simulink library "xrbsComm_r3"  (Simulink 5.1)
libraries: xbsIndex_r3 x775, xrbsComm_r3 x1
(part 2 of 6)

== system xrbsComm_r3/White Gaussian  Noise Generator/Box-Muller1/f/lfsr_41_2 ==
  note: 4-Bit Leap-Forward LFSR G(X) = X^41 + X^3 + 1
  reset : Inport
  Concat : xbsIndex_r3/Concat  explicit_period=off  period=1  dbl_ovrd=off
  Concat1 : xbsIndex_r3/Concat  explicit_period=off  period=1  dbl_ovrd=off
  Concat2 : xbsIndex_r3/Concat  explicit_period=off  period=1  dbl_ovrd=off
  Logical{,1..3} (4 alike) : xbsIndex_r3/Logical  logical_function=XOR  inputs=2  precision=User Defined  arith_type=Unsigned  n_bits=1  bin_pt=0  align_bp=on  latency=0  explicit_period=on  period=-1  en=off  dbl_ovrd=off
      settings: xl_area=[0, 0, 0, 0, 0, 0, 0]
  x : xbsIndex_r3/Register  init=init(1)  reg_only_valid=off  explicit_period=off  period=1  rst=on  en=off  out_en=off  dbl_ovrd=off
      settings: xl_area=[0, 0, 0, 0, 0, 0, 0]
  x1 : Subsystem  mask{init=init(6:4:38)}
  x2 : xbsIndex_r3/Register  init=init(2)  reg_only_valid=off  explicit_period=off  period=1  rst=on  en=off  out_en=off  dbl_ovrd=off
      settings: xl_area=[0, 0, 0, 0, 0, 0, 0]
  x3 : xbsIndex_r3/Register  init=init(3)  reg_only_valid=off  explicit_period=off  period=1  rst=on  en=off  out_en=off  dbl_ovrd=off
      settings: xl_area=[0, 0, 0, 0, 0, 0, 0]
  x4 : xbsIndex_r3/Register  init=init(4)  reg_only_valid=off  explicit_period=off  period=1  rst=on  en=off  out_en=off  dbl_ovrd=off
      settings: xl_area=[0, 0, 0, 0, 0, 0, 0]
  x5 : Subsystem  mask{init=init(5:4:41)}
  x6 : Subsystem  mask{init=init(7:4:39)}
  x7 : Subsystem  mask{init=init(8:4:40)}
  " " : Outport
  wires:
  Logical/1 -> x5/1(" ")
  Logical1/1 -> x1/1(" ")
  Logical2/1 -> x6/1(" ")
  Logical3/1 -> x7/1(" ")
  x5/1(z-10) -> x/1, Logical2/2
  x1/1(z-9) -> x2/1, Logical3/2
  x6/1(z-9) -> x3/1, Logical/2
  x7/1(z-9) -> x4/1
  x/1 -> Logical1/1, Concat/1
  x2/1 -> Concat/2, Logical2/1
  Concat/1 -> Concat2/1
  x3/1 -> Concat1/1, Logical3/1
  x4/1 -> Concat1/2, Logical1/2, Logical/1
  Concat1/1 -> Concat2/2
  Concat2/1 -> " "/1
  reset/1 -> x5/2(reset), x1/2(reset), x6/2(reset), x7/2(reset), x/2, x2/2, x3/2, x4/2

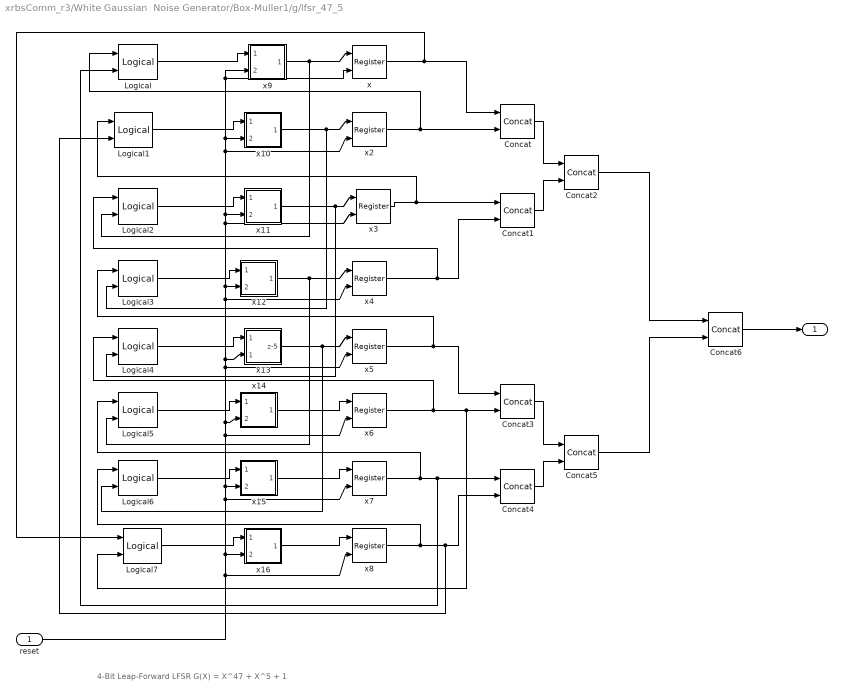
== system xrbsComm_r3/White Gaussian  Noise Generator/Box-Muller1/g/lfsr_47_5 ==
  note: 4-Bit Leap-Forward LFSR G(X) = X^47 + X^5 + 1
  reset : Inport
  Concat{,1..6} (7 alike) : xbsIndex_r3/Concat  explicit_period=off  period=1  dbl_ovrd=off
  Logical{,1..7} (8 alike) : xbsIndex_r3/Logical  logical_function=XOR  inputs=2  precision=User Defined  arith_type=Unsigned  n_bits=1  bin_pt=0  align_bp=on  latency=0  explicit_period=on  period=-1  en=off  dbl_ovrd=off
      settings: xl_area=[0, 0, 0, 0, 0, 0, 0]
  x : xbsIndex_r3/Register  init=init(1)  reg_only_valid=off  explicit_period=off  period=1  rst=on  en=off  out_en=off  dbl_ovrd=off
      settings: xl_area=[0, 0, 0, 0, 0, 0, 0]
  x10 : Subsystem  mask{init=init(10:8:42)}
  x11 : Subsystem  mask{init=init(11:8:43)}
  x12 : Subsystem  mask{init=init(12:8:44)}
  x13 : Subsystem  mask{init=init(13:8:45)}
  x14 : Subsystem  mask{init=init(14:8:46)}
  x15 : Subsystem  mask{init=init(15:8:47)}
  x16 : Subsystem  mask{init=init(16:8:40)}
  x2 : xbsIndex_r3/Register  init=init(2)  reg_only_valid=off  explicit_period=off  period=1  rst=on  en=off  out_en=off  dbl_ovrd=off
      settings: xl_area=[0, 0, 0, 0, 0, 0, 0]
  x3 : xbsIndex_r3/Register  init=init(3)  reg_only_valid=off  explicit_period=off  period=1  rst=on  en=off  out_en=off  dbl_ovrd=off
      settings: xl_area=[0, 0, 0, 0, 0, 0, 0]
  x4 : xbsIndex_r3/Register  init=init(4)  reg_only_valid=off  explicit_period=off  period=1  rst=on  en=off  out_en=off  dbl_ovrd=off
      settings: xl_area=[0, 0, 0, 0, 0, 0, 0]
  x5 : xbsIndex_r3/Register  init=init(5)  reg_only_valid=off  explicit_period=off  period=1  rst=on  en=off  out_en=off  dbl_ovrd=off
      settings: xl_area=[0, 0, 0, 0, 0, 0, 0]
  x6 : xbsIndex_r3/Register  init=init(6)  reg_only_valid=off  explicit_period=off  period=1  rst=on  en=off  out_en=off  dbl_ovrd=off
      settings: xl_area=[0, 0, 0, 0, 0, 0, 0]
  x7 : xbsIndex_r3/Register  init=init(7)  reg_only_valid=off  explicit_period=off  period=1  rst=on  en=off  out_en=off  dbl_ovrd=off
      settings: xl_area=[0, 0, 0, 0, 0, 0, 0]
  x8 : xbsIndex_r3/Register  init=init(8)  reg_only_valid=off  explicit_period=off  period=1  rst=on  en=off  out_en=off  dbl_ovrd=off
      settings: xl_area=[0, 0, 0, 0, 0, 0, 0]
  x9 : Subsystem  mask{init=init(9:8:41)}
  " " : Outport
  wires:
  Logical/1 -> x9/1(" ")
  x9/1(z-5) -> x/1, Logical2/2
  x/1 -> Concat/1, Logical7/1
  x2/1 -> Concat/2, Logical/1
  Concat/1 -> Concat2/1
  x3/1 -> Concat1/1, Logical1/1
  x4/1 -> Concat1/2, Logical2/1
  Concat1/1 -> Concat2/2
  Logical1/1 -> x10/1("  ")
  x10/1(z-5) -> x2/1, Logical3/2
  Logical2/1 -> x11/1(" ")
  x11/1(z-5) -> x3/1, Logical4/2
  Logical3/1 -> x12/1(" ")
  x12/1(z-5) -> x4/1, Logical5/2
  Logical4/1 -> x13/1(" ")
  x13/1(z-5) -> x5/1, Logical6/2
  Logical5/1 -> x14/1(" ")
  x14/1(z-5) -> x6/1
  Logical6/1 -> x15/1(" ")
  x15/1(z-5) -> x7/1
  Logical7/1 -> x16/1(" ")
  x16/1(z-4) -> x8/1
  x6/1 -> Logical4/1, Concat3/2, Logical7/2
  Concat3/1 -> Concat5/1
  Concat4/1 -> Concat5/2
  x5/1 -> Concat3/1, Logical3/1
  x7/1 -> Concat4/1, Logical/2, Logical5/1
  x8/1 -> Concat4/2, Logical1/2, Logical6/1
  Concat2/1 -> Concat6/1
  Concat5/1 -> Concat6/2
  Concat6/1 -> " "/1
  reset/1 -> x9/2(reset), x/2, x10/2(reset), x2/2, x11/2(reset), x3/2, x12/2(reset), x4/2, x13/2(" 1"), x5/2, x14/2(reset), x6/2, x15/2(reset), x7/2, x16/2(reset), x8/2

== system xrbsComm_r3/White Gaussian  Noise Generator/Box-Muller2/fr1/iszero ==
  " " : Inport
  "const " : xbsIndex_r3/Constant  const=0  arith_type=Unsigned  n_bits=4  bin_pt=0  explicit_period=off  period=1  dbl_ovrd=off
  sel1 : xbsIndex_r3/Relational  mode=a=b  latency=1  explicit_period=off  period=1  en=off  dbl_ovrd=off
      settings: xl_area=[0, 0, 0, 0, 0, 0, 0]
  eq : Outport
  wires:
  "const "/1 -> sel1/2
  " "/1 -> sel1/1
  sel1/1 -> eq/1

== system xrbsComm_r3/White Gaussian  Noise Generator/Box-Muller2/fr1/iszero1 ==
  " " : Inport
  Constant1 : xbsIndex_r3/Constant  const=0  arith_type=Unsigned  n_bits=4  bin_pt=0  explicit_period=off  period=1  dbl_ovrd=off
  sel2 : xbsIndex_r3/Relational  mode=a=b  latency=1  explicit_period=off  period=1  en=off  dbl_ovrd=off
      settings: xl_area=[0, 0, 0, 0, 0, 0, 0]
  eq : Outport
  wires:
  Constant1/1 -> sel2/2
  " "/1 -> sel2/1
  sel2/1 -> eq/1

== system xrbsComm_r3/White Gaussian  Noise Generator/Box-Muller2/fr1/iszero2 ==
  " " : Inport
  Constant3 : xbsIndex_r3/Constant  const=0  arith_type=Unsigned  n_bits=4  bin_pt=0  explicit_period=off  period=1  dbl_ovrd=off
  sel3 : xbsIndex_r3/Relational  mode=a=b  latency=1  explicit_period=off  period=1  en=off  dbl_ovrd=off
      settings: xl_area=[0, 0, 0, 0, 0, 0, 0]
  eq : Outport
  wires:
  Constant3/1 -> sel3/2
  " "/1 -> sel3/1
  sel3/1 -> eq/1

== system xrbsComm_r3/White Gaussian  Noise Generator/Box-Muller2/fr1/iszero3 ==
  " " : Inport
  Constant : xbsIndex_r3/Constant  const=0  arith_type=Unsigned  n_bits=4  bin_pt=0  explicit_period=off  period=1  dbl_ovrd=off
  sel4 : xbsIndex_r3/Relational  mode=a=b  latency=1  explicit_period=off  period=1  en=off  dbl_ovrd=off
      settings: xl_area=[0, 0, 0, 0, 0, 0, 0]
  eq : Outport
  wires:
  Constant/1 -> sel4/2
  " "/1 -> sel4/1
  sel4/1 -> eq/1

== system xrbsComm_r3/White Gaussian  Noise Generator/Box-Muller2/fr1/lfsr_17_2 ==
  note: 4-Bit Leap-Forward LFSR G(X) = X^17 + X^3 + 1
  reset : Inport
  Concat : xbsIndex_r3/Concat  explicit_period=off  period=1  dbl_ovrd=off
  Concat1 : xbsIndex_r3/Concat  explicit_period=off  period=1  dbl_ovrd=off
  Concat2 : xbsIndex_r3/Concat  explicit_period=off  period=1  dbl_ovrd=off
  Logical{,1..3} (4 alike) : xbsIndex_r3/Logical  logical_function=XOR  inputs=2  precision=User Defined  arith_type=Unsigned  n_bits=1  bin_pt=0  align_bp=on  latency=0  explicit_period=on  period=-1  en=off  dbl_ovrd=off
      settings: xl_area=[0, 0, 0, 0, 0, 0, 0]
  x : xbsIndex_r3/Register  init=init(1)  reg_only_valid=off  explicit_period=off  period=1  rst=on  en=off  out_en=off  dbl_ovrd=off
      settings: xl_area=[0, 0, 0, 0, 0, 0, 0]
  x1 : Subsystem  mask{init=init(7:4:15)}
  x2 : xbsIndex_r3/Register  init=init(2)  reg_only_valid=off  explicit_period=off  period=1  rst=on  en=off  out_en=off  dbl_ovrd=off
      settings: xl_area=[0, 0, 0, 0, 0, 0, 0]
  x3 : xbsIndex_r3/Register  init=init(3)  reg_only_valid=off  explicit_period=off  period=1  rst=on  en=off  out_en=off  dbl_ovrd=off
      settings: xl_area=[0, 0, 0, 0, 0, 0, 0]
  x4 : xbsIndex_r3/Register  init=init(4)  reg_only_valid=off  explicit_period=off  period=1  rst=on  en=off  out_en=off  dbl_ovrd=off
      settings: xl_area=[0, 0, 0, 0, 0, 0, 0]
  x5 : Subsystem  mask{init=init(5:4:17)}
  x6 : Subsystem  mask{init=init(6:4:14)}
  x7 : Subsystem  mask{init=init(8:4:16)}
  " " : Outport
  wires:
  Logical/1 -> x5/1(" ")
  Logical1/1 -> x6/1(" ")
  Logical2/1 -> x1/1(" ")
  Logical3/1 -> x7/1(" ")
  x5/1(z-4) -> x/1, Logical2/2
  x6/1(z-3) -> x2/1, Logical3/2
  x1/1(z-3) -> x3/1, Logical/2
  x7/1(z-3) -> x4/1
  x/1 -> Logical1/1, Concat/1
  x2/1 -> Concat/2, Logical2/1
  Concat/1 -> Concat2/1
  x3/1 -> Concat1/1, Logical3/1
  x4/1 -> Concat1/2, Logical1/2, Logical/1
  Concat1/1 -> Concat2/2
  Concat2/1 -> " "/1
  reset/1 -> x5/2(reset), x6/2(" reset"), x1/2(" reset"), x7/2(reset), x/2, x2/2, x3/2, x4/2

== system xrbsComm_r3/White Gaussian  Noise Generator/Box-Muller2/fr1/lfsr_25_2 ==
  note: 4-Bit Leap-Forward LFSR G(X) = X^25 + X^3 + 1
  " reset" : Inport
  Concat : xbsIndex_r3/Concat  explicit_period=off  period=1  dbl_ovrd=off
  Concat1 : xbsIndex_r3/Concat  explicit_period=off  period=1  dbl_ovrd=off
  Concat2 : xbsIndex_r3/Concat  explicit_period=off  period=1  dbl_ovrd=off
  Logical{,1..3} (4 alike) : xbsIndex_r3/Logical  logical_function=XOR  inputs=2  precision=User Defined  arith_type=Unsigned  n_bits=1  bin_pt=0  align_bp=on  latency=0  explicit_period=on  period=-1  en=off  dbl_ovrd=off
      settings: xl_area=[0, 0, 0, 0, 0, 0, 0]
  x : xbsIndex_r3/Register  init=init(1)  reg_only_valid=off  explicit_period=off  period=1  rst=on  en=off  out_en=off  dbl_ovrd=off
      settings: xl_area=[0, 0, 0, 0, 0, 0, 0]
  x1 : Subsystem  mask{init=init(7:4:23)}
  x2 : xbsIndex_r3/Register  init=init(2)  reg_only_valid=off  explicit_period=off  period=1  rst=on  en=off  out_en=off  dbl_ovrd=off
      settings: xl_area=[0, 0, 0, 0, 0, 0, 0]
  x3 : xbsIndex_r3/Register  init=init(3)  reg_only_valid=off  explicit_period=off  period=1  rst=on  en=off  out_en=off  dbl_ovrd=off
      settings: xl_area=[0, 0, 0, 0, 0, 0, 0]
  x4 : xbsIndex_r3/Register  init=init(4)  reg_only_valid=off  explicit_period=off  period=1  rst=on  en=off  out_en=off  dbl_ovrd=off
      settings: xl_area=[0, 0, 0, 0, 0, 0, 0]
  x5 : Subsystem  mask{init=init(5:4:25)}
  x6 : Subsystem  mask{init=init(6:4:22)}
  x7 : Subsystem  mask{init=init(8:4:24)}
  " " : Outport
  wires:
  Concat2/1 -> " "/1
  Concat1/1 -> Concat2/2
  x4/1 -> Logical/1, Logical1/2, Concat1/2
  x3/1 -> Logical3/1, Concat1/1
  Concat/1 -> Concat2/1
  x/1 -> Concat/1, Logical1/1
  x7/1(z-5) -> x4/1
  x1/1(z-5) -> Logical/2, x3/1
  x6/1(z-5) -> Logical3/2, x2/1
  x5/1(z-6) -> Logical2/2, x/1
  Logical3/1 -> x7/1(" ")
  Logical2/1 -> x1/1(" ")
  Logical1/1 -> x6/1(" ")
  Logical/1 -> x5/1(" ")
  " reset"/1 -> x7/2(reset), x1/2(reset), x6/2(reset), x5/2(reset), x/2, x2/2, x3/2, x4/2
  x2/1 -> Concat/2, Logical2/1

== system xrbsComm_r3/White Gaussian  Noise Generator/Box-Muller2/fr1/lfsr_29_2 ==
  note: 4-Bit Leap-Forward LFSR G(X) = X^29 + X^2 + 1
  reset : Inport
  Concat : xbsIndex_r3/Concat  explicit_period=off  period=1  dbl_ovrd=off
  Concat1 : xbsIndex_r3/Concat  explicit_period=off  period=1  dbl_ovrd=off
  Concat2 : xbsIndex_r3/Concat  explicit_period=off  period=1  dbl_ovrd=off
  Logical{,1..3} (4 alike) : xbsIndex_r3/Logical  logical_function=XOR  inputs=2  precision=User Defined  arith_type=Unsigned  n_bits=1  bin_pt=0  align_bp=on  latency=0  explicit_period=on  period=-1  en=off  dbl_ovrd=off
      settings: xl_area=[0, 0, 0, 0, 0, 0, 0]
  x : xbsIndex_r3/Register  init=init(1)  reg_only_valid=off  explicit_period=off  period=1  rst=on  en=off  out_en=off  dbl_ovrd=off
      settings: xl_area=[0, 0, 0, 0, 0, 0, 0]
  x2 : xbsIndex_r3/Register  init=init(2)  reg_only_valid=off  explicit_period=off  period=1  rst=on  en=off  out_en=off  dbl_ovrd=off
      settings: xl_area=[0, 0, 0, 0, 0, 0, 0]
  x3 : xbsIndex_r3/Register  init=init(3)  reg_only_valid=off  explicit_period=off  period=1  rst=on  en=off  out_en=off  dbl_ovrd=off
      settings: xl_area=[0, 0, 0, 0, 0, 0, 0]
  x4 : xbsIndex_r3/Register  init=init(4)  reg_only_valid=off  explicit_period=off  period=1  rst=on  en=off  out_en=off  dbl_ovrd=off
      settings: xl_area=[0, 0, 0, 0, 0, 0, 0]
  x5 : Subsystem  mask{init=init(5:4:29)}
  x6 : Subsystem  mask{init=init(6:4:26)}
  x7 : Subsystem  mask{init=init(7:4:27)}
  x8 : Subsystem  mask{init=init(8:4:28)}
  " " : Outport
  wires:
  Logical/1 -> x5/1(" ")
  Logical1/1 -> x6/1(" ")
  Logical2/1 -> x7/1(" ")
  Logical3/1 -> x8/1(" ")
  x5/1(z-7) -> x/1, Logical3/2
  x6/1(z-6) -> x2/1, Logical/2
  x7/1(z-6) -> x3/1
  x8/1(z-6) -> x4/1
  x/1 -> Logical1/1, Concat/1
  x2/1 -> Concat/2, Logical2/1
  Concat/1 -> Concat2/1
  x3/1 -> Concat1/1, Logical1/2, Logical3/1
  x4/1 -> Concat1/2, Logical2/2, Logical/1
  Concat1/1 -> Concat2/2
  Concat2/1 -> " "/1
  reset/1 -> x8/2(reset), x7/2(reset), x6/2(reset), x5/2(reset), x/2, x2/2, x3/2, x4/2

== system xrbsComm_r3/White Gaussian  Noise Generator/Box-Muller2/fr1/lfsr_31_2 ==
  note: 4-Bit Leap-Forward LFSR G(X) = X^31 + X^3 + 1
  reset : Inport
  Concat : xbsIndex_r3/Concat  explicit_period=off  period=1  dbl_ovrd=off
  Concat1 : xbsIndex_r3/Concat  explicit_period=off  period=1  dbl_ovrd=off
  Concat2 : xbsIndex_r3/Concat  explicit_period=off  period=1  dbl_ovrd=off
  Logical{,1..3} (4 alike) : xbsIndex_r3/Logical  logical_function=XOR  inputs=2  precision=User Defined  arith_type=Unsigned  n_bits=1  bin_pt=0  align_bp=on  latency=0  explicit_period=on  period=-1  en=off  dbl_ovrd=off
      settings: xl_area=[0, 0, 0, 0, 0, 0, 0]
  x : xbsIndex_r3/Register  init=init(1)  reg_only_valid=off  explicit_period=off  period=1  rst=on  en=off  out_en=off  dbl_ovrd=off
      settings: xl_area=[0, 0, 0, 0, 0, 0, 0]
  x2 : xbsIndex_r3/Register  init=init(2)  reg_only_valid=off  explicit_period=off  period=1  rst=on  en=off  out_en=off  dbl_ovrd=off
      settings: xl_area=[0, 0, 0, 0, 0, 0, 0]
  x3 : xbsIndex_r3/Register  init=init(3)  reg_only_valid=off  explicit_period=off  period=1  rst=on  en=off  out_en=off  dbl_ovrd=off
      settings: xl_area=[0, 0, 0, 0, 0, 0, 0]
  x4 : xbsIndex_r3/Register  init=init(4)  reg_only_valid=off  explicit_period=off  period=1  rst=on  en=off  out_en=off  dbl_ovrd=off
      settings: xl_area=[0, 0, 0, 0, 0, 0, 0]
  x5 : Subsystem  mask{init=init(5:4:29)}
  x6 : Subsystem  mask{init=init(6:4:30)}
  x7 : Subsystem  mask{init=init(7:4:31)}
  x8 : Subsystem  mask{init=init(8:4:28)}
  " " : Outport
  wires:
  Logical/1 -> x5/1(" ")
  Logical1/1 -> x6/1(" ")
  Logical2/1 -> x7/1(" ")
  Logical3/1 -> x8/1(" ")
  x5/1(z-7) -> Logical/1, x/1
  x6/1(z-7) -> Logical1/1, x2/1
  x7/1(z-7) -> x3/1, Logical2/1
  x8/1(z-6) -> x4/1
  x/1 -> Concat/1, Logical3/1
  x2/1 -> Concat/2, Logical/2
  Concat/1 -> Concat2/1
  x3/1 -> Concat1/1, Logical1/2
  x4/1 -> Logical3/2, Concat1/2, Logical2/2
  Concat1/1 -> Concat2/2
  Concat2/1 -> " "/1
  reset/1 -> x7/2(reset), x5/2(reset), x6/2(reset), x8/2(reset), x/2, x2/2, x3/2, x4/2

== system xrbsComm_r3/White Gaussian  Noise Generator/Box-Muller2/fr1/lfsr_41_2 ==
  note: 4-Bit Leap-Forward LFSR G(X) = X^41 + X^3 + 1
  reset : Inport
  Concat : xbsIndex_r3/Concat  explicit_period=off  period=1  dbl_ovrd=off
  Concat1 : xbsIndex_r3/Concat  explicit_period=off  period=1  dbl_ovrd=off
  Concat2 : xbsIndex_r3/Concat  explicit_period=off  period=1  dbl_ovrd=off
  Logical{,1..3} (4 alike) : xbsIndex_r3/Logical  logical_function=XOR  inputs=2  precision=User Defined  arith_type=Unsigned  n_bits=1  bin_pt=0  align_bp=on  latency=0  explicit_period=on  period=-1  en=off  dbl_ovrd=off
      settings: xl_area=[0, 0, 0, 0, 0, 0, 0]
  x : xbsIndex_r3/Register  init=init(1)  reg_only_valid=off  explicit_period=off  period=1  rst=on  en=off  out_en=off  dbl_ovrd=off
      settings: xl_area=[0, 0, 0, 0, 0, 0, 0]
  x1 : Subsystem  mask{init=init(6:4:38)}
  x2 : xbsIndex_r3/Register  init=init(2)  reg_only_valid=off  explicit_period=off  period=1  rst=on  en=off  out_en=off  dbl_ovrd=off
      settings: xl_area=[0, 0, 0, 0, 0, 0, 0]
  x3 : xbsIndex_r3/Register  init=init(3)  reg_only_valid=off  explicit_period=off  period=1  rst=on  en=off  out_en=off  dbl_ovrd=off
      settings: xl_area=[0, 0, 0, 0, 0, 0, 0]
  x4 : xbsIndex_r3/Register  init=init(4)  reg_only_valid=off  explicit_period=off  period=1  rst=on  en=off  out_en=off  dbl_ovrd=off
      settings: xl_area=[0, 0, 0, 0, 0, 0, 0]
  x5 : Subsystem  mask{init=init(5:4:41)}
  x6 : Subsystem  mask{init=init(7:4:39)}
  x7 : Subsystem  mask{init=init(8:4:40)}
  " " : Outport
  wires:
  Logical/1 -> x5/1(" ")
  Logical1/1 -> x1/1(" ")
  Logical2/1 -> x6/1(" ")
  Logical3/1 -> x7/1(" ")
  x5/1(z-10) -> x/1, Logical2/2
  x1/1(z-9) -> x2/1, Logical3/2
  x6/1(z-9) -> x3/1, Logical/2
  x7/1(z-9) -> x4/1
  x/1 -> Logical1/1, Concat/1
  x2/1 -> Concat/2, Logical2/1
  Concat/1 -> Concat2/1
  x3/1 -> Concat1/1, Logical3/1
  x4/1 -> Concat1/2, Logical1/2, Logical/1
  Concat1/1 -> Concat2/2
  Concat2/1 -> " "/1
  reset/1 -> x5/2(reset), x1/2(reset), x6/2(reset), x7/2(reset), x/2, x2/2, x3/2, x4/2

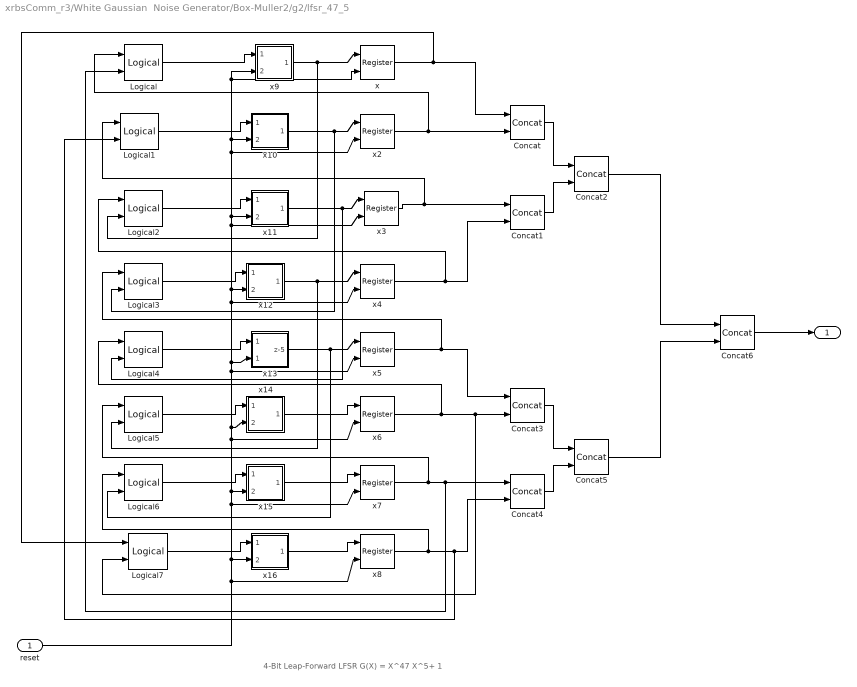
== system xrbsComm_r3/White Gaussian  Noise Generator/Box-Muller2/g2/lfsr_47_5 ==
  note: 4-Bit Leap-Forward LFSR G(X) = X^47 X^5+ 1
  reset : Inport
  Concat{,1..6} (7 alike) : xbsIndex_r3/Concat  explicit_period=off  period=1  dbl_ovrd=off
  Logical{,1..7} (8 alike) : xbsIndex_r3/Logical  logical_function=XOR  inputs=2  precision=User Defined  arith_type=Unsigned  n_bits=1  bin_pt=0  align_bp=on  latency=0  explicit_period=on  period=-1  en=off  dbl_ovrd=off
      settings: xl_area=[0, 0, 0, 0, 0, 0, 0]
  x : xbsIndex_r3/Register  init=init(1)  reg_only_valid=off  explicit_period=off  period=1  rst=on  en=off  out_en=off  dbl_ovrd=off
      settings: xl_area=[0, 0, 0, 0, 0, 0, 0]
  x10 : Subsystem  mask{init=init(10:8:42)}
  x11 : Subsystem  mask{init=init(11:8:43)}
  x12 : Subsystem  mask{init=init(12:8:44)}
  x13 : Subsystem  mask{init=init(13:8:45)}
  x14 : Subsystem  mask{init=init(14:8:46)}
  x15 : Subsystem  mask{init=init(15:8:47)}
  x16 : Subsystem  mask{init=init(16:8:40)}
  x2 : xbsIndex_r3/Register  init=init(2)  reg_only_valid=off  explicit_period=off  period=1  rst=on  en=off  out_en=off  dbl_ovrd=off
      settings: xl_area=[0, 0, 0, 0, 0, 0, 0]
  x3 : xbsIndex_r3/Register  init=init(3)  reg_only_valid=off  explicit_period=off  period=1  rst=on  en=off  out_en=off  dbl_ovrd=off
      settings: xl_area=[0, 0, 0, 0, 0, 0, 0]
  x4 : xbsIndex_r3/Register  init=init(4)  reg_only_valid=off  explicit_period=off  period=1  rst=on  en=off  out_en=off  dbl_ovrd=off
      settings: xl_area=[0, 0, 0, 0, 0, 0, 0]
  x5 : xbsIndex_r3/Register  init=init(5)  reg_only_valid=off  explicit_period=off  period=1  rst=on  en=off  out_en=off  dbl_ovrd=off
      settings: xl_area=[0, 0, 0, 0, 0, 0, 0]
  x6 : xbsIndex_r3/Register  init=init(6)  reg_only_valid=off  explicit_period=off  period=1  rst=on  en=off  out_en=off  dbl_ovrd=off
      settings: xl_area=[0, 0, 0, 0, 0, 0, 0]
  x7 : xbsIndex_r3/Register  init=init(7)  reg_only_valid=off  explicit_period=off  period=1  rst=on  en=off  out_en=off  dbl_ovrd=off
      settings: xl_area=[0, 0, 0, 0, 0, 0, 0]
  x8 : xbsIndex_r3/Register  init=init(8)  reg_only_valid=off  explicit_period=off  period=1  rst=on  en=off  out_en=off  dbl_ovrd=off
      settings: xl_area=[0, 0, 0, 0, 0, 0, 0]
  x9 : Subsystem  mask{init=init(9:8:41)}
  " " : Outport
  wires:
  Logical/1 -> x9/1(" ")
  x9/1(z-5) -> x/1, Logical2/2
  x/1 -> Concat/1, Logical7/1
  x2/1 -> Concat/2, Logical/1
  Concat/1 -> Concat2/1
  x3/1 -> Concat1/1, Logical1/1
  x4/1 -> Concat1/2, Logical2/1
  Concat1/1 -> Concat2/2
  Logical1/1 -> x10/1("  ")
  x10/1(z-5) -> x2/1, Logical3/2
  Logical2/1 -> x11/1(" ")
  x11/1(z-5) -> x3/1, Logical4/2
  Logical3/1 -> x12/1(" ")
  x12/1(z-5) -> x4/1, Logical5/2
  Logical4/1 -> x13/1(" ")
  x13/1(z-5) -> x5/1, Logical6/2
  Logical5/1 -> x14/1(" ")
  x14/1(z-5) -> x6/1
  Logical6/1 -> x15/1(" ")
  x15/1(z-5) -> x7/1
  Logical7/1 -> x16/1(" ")
  x16/1(z-4) -> x8/1
  x6/1 -> Logical4/1, Concat3/2, Logical7/2
  Concat3/1 -> Concat5/1
  Concat4/1 -> Concat5/2
  x5/1 -> Concat3/1, Logical3/1
  x7/1 -> Concat4/1, Logical/2, Logical5/1
  x8/1 -> Concat4/2, Logical1/2, Logical6/1
  Concat2/1 -> Concat6/1
  Concat5/1 -> Concat6/2
  Concat6/1 -> " "/1
  reset/1 -> x9/2(reset), x/2, x10/2(reset), x2/2, x11/2(reset), x3/2, x12/2(reset), x4/2, x13/2(" 1"), x5/2, x14/2(reset), x6/2, x15/2(reset), x7/2, x16/2(reset), x8/2

== system xrbsComm_r3/White Gaussian  Noise Generator/Box-Muller3/fr1/iszero ==
  " " : Inport
  "const " : xbsIndex_r3/Constant  const=0  arith_type=Unsigned  n_bits=4  bin_pt=0  explicit_period=off  period=1  dbl_ovrd=off
  sel1 : xbsIndex_r3/Relational  mode=a=b  latency=1  explicit_period=off  period=1  en=off  dbl_ovrd=off
      settings: xl_area=[0, 0, 0, 0, 0, 0, 0]
  eq : Outport
  wires:
  "const "/1 -> sel1/2
  " "/1 -> sel1/1
  sel1/1 -> eq/1

== system xrbsComm_r3/White Gaussian  Noise Generator/Box-Muller3/fr1/iszero1 ==
  " " : Inport
  Constant1 : xbsIndex_r3/Constant  const=0  arith_type=Unsigned  n_bits=4  bin_pt=0  explicit_period=off  period=1  dbl_ovrd=off
  sel2 : xbsIndex_r3/Relational  mode=a=b  latency=1  explicit_period=off  period=1  en=off  dbl_ovrd=off
      settings: xl_area=[0, 0, 0, 0, 0, 0, 0]
  eq : Outport
  wires:
  Constant1/1 -> sel2/2
  " "/1 -> sel2/1
  sel2/1 -> eq/1

== system xrbsComm_r3/White Gaussian  Noise Generator/Box-Muller3/fr1/iszero2 ==
  " " : Inport
  Constant3 : xbsIndex_r3/Constant  const=0  arith_type=Unsigned  n_bits=4  bin_pt=0  explicit_period=off  period=1  dbl_ovrd=off
  sel3 : xbsIndex_r3/Relational  mode=a=b  latency=1  explicit_period=off  period=1  en=off  dbl_ovrd=off
      settings: xl_area=[0, 0, 0, 0, 0, 0, 0]
  eq : Outport
  wires:
  Constant3/1 -> sel3/2
  " "/1 -> sel3/1
  sel3/1 -> eq/1

== system xrbsComm_r3/White Gaussian  Noise Generator/Box-Muller3/fr1/iszero3 ==
  " " : Inport
  Constant : xbsIndex_r3/Constant  const=0  arith_type=Unsigned  n_bits=4  bin_pt=0  explicit_period=off  period=1  dbl_ovrd=off
  sel4 : xbsIndex_r3/Relational  mode=a=b  latency=1  explicit_period=off  period=1  en=off  dbl_ovrd=off
      settings: xl_area=[0, 0, 0, 0, 0, 0, 0]
  eq : Outport
  wires:
  Constant/1 -> sel4/2
  " "/1 -> sel4/1
  sel4/1 -> eq/1

== system xrbsComm_r3/White Gaussian  Noise Generator/Box-Muller3/fr1/lfsr_17_2 ==
  note: 4-Bit Leap-Forward LFSR G(X) = X^17 + X^3 + 1
  reset : Inport
  Concat : xbsIndex_r3/Concat  explicit_period=off  period=1  dbl_ovrd=off
  Concat1 : xbsIndex_r3/Concat  explicit_period=off  period=1  dbl_ovrd=off
  Concat2 : xbsIndex_r3/Concat  explicit_period=off  period=1  dbl_ovrd=off
  Logical{,1..3} (4 alike) : xbsIndex_r3/Logical  logical_function=XOR  inputs=2  precision=User Defined  arith_type=Unsigned  n_bits=1  bin_pt=0  align_bp=on  latency=0  explicit_period=on  period=-1  en=off  dbl_ovrd=off
      settings: xl_area=[0, 0, 0, 0, 0, 0, 0]
  x : xbsIndex_r3/Register  init=init(1)  reg_only_valid=off  explicit_period=off  period=1  rst=on  en=off  out_en=off  dbl_ovrd=off
      settings: xl_area=[0, 0, 0, 0, 0, 0, 0]
  x1 : Subsystem  mask{init=init(7:4:15)}
  x2 : xbsIndex_r3/Register  init=init(2)  reg_only_valid=off  explicit_period=off  period=1  rst=on  en=off  out_en=off  dbl_ovrd=off
      settings: xl_area=[0, 0, 0, 0, 0, 0, 0]
  x3 : xbsIndex_r3/Register  init=init(3)  reg_only_valid=off  explicit_period=off  period=1  rst=on  en=off  out_en=off  dbl_ovrd=off
      settings: xl_area=[0, 0, 0, 0, 0, 0, 0]
  x4 : xbsIndex_r3/Register  init=init(4)  reg_only_valid=off  explicit_period=off  period=1  rst=on  en=off  out_en=off  dbl_ovrd=off
      settings: xl_area=[0, 0, 0, 0, 0, 0, 0]
  x5 : Subsystem  mask{init=init(5:4:17)}
  x6 : Subsystem  mask{init=init(6:4:14)}
  x7 : Subsystem  mask{init=init(8:4:16)}
  " " : Outport
  wires:
  Logical/1 -> x5/1(" ")
  Logical1/1 -> x6/1(" ")
  Logical2/1 -> x1/1(" ")
  Logical3/1 -> x7/1(" ")
  x5/1(z-4) -> x/1, Logical2/2
  x6/1(z-3) -> x2/1, Logical3/2
  x1/1(z-3) -> x3/1, Logical/2
  x7/1(z-3) -> x4/1
  x/1 -> Logical1/1, Concat/1
  x2/1 -> Concat/2, Logical2/1
  Concat/1 -> Concat2/1
  x3/1 -> Concat1/1, Logical3/1
  x4/1 -> Concat1/2, Logical1/2, Logical/1
  Concat1/1 -> Concat2/2
  Concat2/1 -> " "/1
  reset/1 -> x5/2(reset), x6/2(" reset"), x1/2(" reset"), x7/2(reset), x/2, x2/2, x3/2, x4/2

== system xrbsComm_r3/White Gaussian  Noise Generator/Box-Muller3/fr1/lfsr_25_2 ==
  note: 4-Bit Leap-Forward LFSR G(X) = X^25 + X^3 + 1
  " reset" : Inport
  Concat : xbsIndex_r3/Concat  explicit_period=off  period=1  dbl_ovrd=off
  Concat1 : xbsIndex_r3/Concat  explicit_period=off  period=1  dbl_ovrd=off
  Concat2 : xbsIndex_r3/Concat  explicit_period=off  period=1  dbl_ovrd=off
  Logical{,1..3} (4 alike) : xbsIndex_r3/Logical  logical_function=XOR  inputs=2  precision=User Defined  arith_type=Unsigned  n_bits=1  bin_pt=0  align_bp=on  latency=0  explicit_period=on  period=-1  en=off  dbl_ovrd=off
      settings: xl_area=[0, 0, 0, 0, 0, 0, 0]
  x : xbsIndex_r3/Register  init=init(1)  reg_only_valid=off  explicit_period=off  period=1  rst=on  en=off  out_en=off  dbl_ovrd=off
      settings: xl_area=[0, 0, 0, 0, 0, 0, 0]
  x1 : Subsystem  mask{init=init(7:4:23)}
  x2 : xbsIndex_r3/Register  init=init(2)  reg_only_valid=off  explicit_period=off  period=1  rst=on  en=off  out_en=off  dbl_ovrd=off
      settings: xl_area=[0, 0, 0, 0, 0, 0, 0]
  x3 : xbsIndex_r3/Register  init=init(3)  reg_only_valid=off  explicit_period=off  period=1  rst=on  en=off  out_en=off  dbl_ovrd=off
      settings: xl_area=[0, 0, 0, 0, 0, 0, 0]
  x4 : xbsIndex_r3/Register  init=init(4)  reg_only_valid=off  explicit_period=off  period=1  rst=on  en=off  out_en=off  dbl_ovrd=off
      settings: xl_area=[0, 0, 0, 0, 0, 0, 0]
  x5 : Subsystem  mask{init=init(5:4:25)}
  x6 : Subsystem  mask{init=init(6:4:22)}
  x7 : Subsystem  mask{init=init(8:4:24)}
  " " : Outport
  wires:
  Concat2/1 -> " "/1
  Concat1/1 -> Concat2/2
  x4/1 -> Logical/1, Logical1/2, Concat1/2
  x3/1 -> Logical3/1, Concat1/1
  Concat/1 -> Concat2/1
  x2/1 -> Logical2/1, Concat/2
  x/1 -> Concat/1, Logical1/1
  x7/1(z-5) -> x4/1
  x1/1(z-5) -> Logical/2, x3/1
  x6/1(z-5) -> Logical3/2, x2/1
  x5/1(z-6) -> Logical2/2, x/1
  Logical3/1 -> x7/1(" ")
  Logical2/1 -> x1/1(" ")
  Logical1/1 -> x6/1(" ")
  Logical/1 -> x5/1(" ")
  " reset"/1 -> x7/2(reset), x1/2(reset), x6/2(reset), x5/2(reset), x/2, x2/2, x3/2, x4/2

== system xrbsComm_r3/White Gaussian  Noise Generator/Box-Muller3/fr1/lfsr_29_2 ==
  note: 4-Bit Leap-Forward LFSR G(X) = X^29 + X^2 + 1
  reset : Inport
  Concat : xbsIndex_r3/Concat  explicit_period=off  period=1  dbl_ovrd=off
  Concat1 : xbsIndex_r3/Concat  explicit_period=off  period=1  dbl_ovrd=off
  Concat2 : xbsIndex_r3/Concat  explicit_period=off  period=1  dbl_ovrd=off
  Logical{,1..3} (4 alike) : xbsIndex_r3/Logical  logical_function=XOR  inputs=2  precision=User Defined  arith_type=Unsigned  n_bits=1  bin_pt=0  align_bp=on  latency=0  explicit_period=on  period=-1  en=off  dbl_ovrd=off
      settings: xl_area=[0, 0, 0, 0, 0, 0, 0]
  x : xbsIndex_r3/Register  init=init(1)  reg_only_valid=off  explicit_period=off  period=1  rst=on  en=off  out_en=off  dbl_ovrd=off
      settings: xl_area=[0, 0, 0, 0, 0, 0, 0]
  x2 : xbsIndex_r3/Register  init=init(2)  reg_only_valid=off  explicit_period=off  period=1  rst=on  en=off  out_en=off  dbl_ovrd=off
      settings: xl_area=[0, 0, 0, 0, 0, 0, 0]
  x3 : xbsIndex_r3/Register  init=init(3)  reg_only_valid=off  explicit_period=off  period=1  rst=on  en=off  out_en=off  dbl_ovrd=off
      settings: xl_area=[0, 0, 0, 0, 0, 0, 0]
  x4 : xbsIndex_r3/Register  init=init(4)  reg_only_valid=off  explicit_period=off  period=1  rst=on  en=off  out_en=off  dbl_ovrd=off
      settings: xl_area=[0, 0, 0, 0, 0, 0, 0]
  x5 : Subsystem  mask{init=init(5:4:29)}
  x6 : Subsystem  mask{init=init(6:4:26)}
  x7 : Subsystem  mask{init=init(7:4:27)}
  x8 : Subsystem  mask{init=init(8:4:28)}
  " " : Outport
  wires:
  Logical/1 -> x5/1(" ")
  Logical1/1 -> x6/1(" ")
  Logical2/1 -> x7/1(" ")
  Logical3/1 -> x8/1(" ")
  x5/1(z-7) -> x/1, Logical3/2
  x6/1(z-6) -> x2/1, Logical/2
  x7/1(z-6) -> x3/1
  x8/1(z-6) -> x4/1
  x/1 -> Logical1/1, Concat/1
  x2/1 -> Concat/2, Logical2/1
  Concat/1 -> Concat2/1
  x3/1 -> Concat1/1, Logical1/2, Logical3/1
  x4/1 -> Concat1/2, Logical2/2, Logical/1
  Concat1/1 -> Concat2/2
  Concat2/1 -> " "/1
  reset/1 -> x8/2(reset), x7/2(reset), x6/2(reset), x5/2(reset), x/2, x2/2, x3/2, x4/2

== system xrbsComm_r3/White Gaussian  Noise Generator/Box-Muller3/fr1/lfsr_31_2 ==
  note: 4-Bit Leap-Forward LFSR G(X) = X^31 + X^3 + 1
  reset : Inport
  Concat : xbsIndex_r3/Concat  explicit_period=off  period=1  dbl_ovrd=off
  Concat1 : xbsIndex_r3/Concat  explicit_period=off  period=1  dbl_ovrd=off
  Concat2 : xbsIndex_r3/Concat  explicit_period=off  period=1  dbl_ovrd=off
  Logical{,1..3} (4 alike) : xbsIndex_r3/Logical  logical_function=XOR  inputs=2  precision=User Defined  arith_type=Unsigned  n_bits=1  bin_pt=0  align_bp=on  latency=0  explicit_period=on  period=-1  en=off  dbl_ovrd=off
      settings: xl_area=[0, 0, 0, 0, 0, 0, 0]
  x : xbsIndex_r3/Register  init=init(1)  reg_only_valid=off  explicit_period=off  period=1  rst=on  en=off  out_en=off  dbl_ovrd=off
      settings: xl_area=[0, 0, 0, 0, 0, 0, 0]
  x2 : xbsIndex_r3/Register  init=init(2)  reg_only_valid=off  explicit_period=off  period=1  rst=on  en=off  out_en=off  dbl_ovrd=off
      settings: xl_area=[0, 0, 0, 0, 0, 0, 0]
  x3 : xbsIndex_r3/Register  init=init(3)  reg_only_valid=off  explicit_period=off  period=1  rst=on  en=off  out_en=off  dbl_ovrd=off
      settings: xl_area=[0, 0, 0, 0, 0, 0, 0]
  x4 : xbsIndex_r3/Register  init=init(4)  reg_only_valid=off  explicit_period=off  period=1  rst=on  en=off  out_en=off  dbl_ovrd=off
      settings: xl_area=[0, 0, 0, 0, 0, 0, 0]
  x5 : Subsystem  mask{init=init(5:4:29)}
  x6 : Subsystem  mask{init=init(6:4:30)}
  x7 : Subsystem  mask{init=init(7:4:31)}
  x8 : Subsystem  mask{init=init(8:4:28)}
  " " : Outport
  wires:
  Logical/1 -> x5/1(" ")
  Logical1/1 -> x6/1(" ")
  Logical2/1 -> x7/1(" ")
  Logical3/1 -> x8/1(" ")
  x5/1(z-7) -> Logical/1, x/1
  x6/1(z-7) -> Logical1/1, x2/1
  x7/1(z-7) -> x3/1, Logical2/1
  x8/1(z-6) -> x4/1
  x/1 -> Concat/1, Logical3/1
  x2/1 -> Concat/2, Logical/2
  Concat/1 -> Concat2/1
  x3/1 -> Concat1/1, Logical1/2
  x4/1 -> Logical2/2, Concat1/2, Logical3/2
  Concat1/1 -> Concat2/2
  Concat2/1 -> " "/1
  reset/1 -> x/2, x2/2, x3/2, x4/2, x5/2(reset), x6/2(reset), x7/2(reset), x8/2(reset)

== system xrbsComm_r3/White Gaussian  Noise Generator/Box-Muller3/fr1/lfsr_41_2 ==
  note: 4-Bit Leap-Forward LFSR G(X) = X^41 + X^3 + 1
  reset : Inport
  Concat : xbsIndex_r3/Concat  explicit_period=off  period=1  dbl_ovrd=off
  Concat1 : xbsIndex_r3/Concat  explicit_period=off  period=1  dbl_ovrd=off
  Concat2 : xbsIndex_r3/Concat  explicit_period=off  period=1  dbl_ovrd=off
  Logical{,1..3} (4 alike) : xbsIndex_r3/Logical  logical_function=XOR  inputs=2  precision=User Defined  arith_type=Unsigned  n_bits=1  bin_pt=0  align_bp=on  latency=0  explicit_period=on  period=-1  en=off  dbl_ovrd=off
      settings: xl_area=[0, 0, 0, 0, 0, 0, 0]
  x : xbsIndex_r3/Register  init=init(1)  reg_only_valid=off  explicit_period=off  period=1  rst=on  en=off  out_en=off  dbl_ovrd=off
      settings: xl_area=[0, 0, 0, 0, 0, 0, 0]
  x1 : Subsystem  mask{init=init(6:4:38)}
  x2 : xbsIndex_r3/Register  init=init(2)  reg_only_valid=off  explicit_period=off  period=1  rst=on  en=off  out_en=off  dbl_ovrd=off
      settings: xl_area=[0, 0, 0, 0, 0, 0, 0]
  x3 : xbsIndex_r3/Register  init=init(3)  reg_only_valid=off  explicit_period=off  period=1  rst=on  en=off  out_en=off  dbl_ovrd=off
      settings: xl_area=[0, 0, 0, 0, 0, 0, 0]
  x4 : xbsIndex_r3/Register  init=init(4)  reg_only_valid=off  explicit_period=off  period=1  rst=on  en=off  out_en=off  dbl_ovrd=off
      settings: xl_area=[0, 0, 0, 0, 0, 0, 0]
  x5 : Subsystem  mask{init=init(5:4:41)}
  x6 : Subsystem  mask{init=init(7:4:39)}
  x7 : Subsystem  mask{init=init(8:4:40)}
  " " : Outport
  wires:
  Logical/1 -> x5/1(" ")
  Logical1/1 -> x1/1(" ")
  Logical2/1 -> x6/1(" ")
  Logical3/1 -> x7/1(" ")
  x5/1(z-10) -> x/1, Logical2/2
  x1/1(z-9) -> x2/1, Logical3/2
  x6/1(z-9) -> x3/1, Logical/2
  x7/1(z-9) -> x4/1
  x/1 -> Logical1/1, Concat/1
  x2/1 -> Concat/2, Logical2/1
  Concat/1 -> Concat2/1
  x3/1 -> Concat1/1, Logical3/1
  x4/1 -> Concat1/2, Logical/1, Logical1/2
  Concat1/1 -> Concat2/2
  Concat2/1 -> " "/1
  reset/1 -> x5/2(reset), x1/2(reset), x6/2(reset), x7/2(reset), x/2, x2/2, x3/2, x4/2

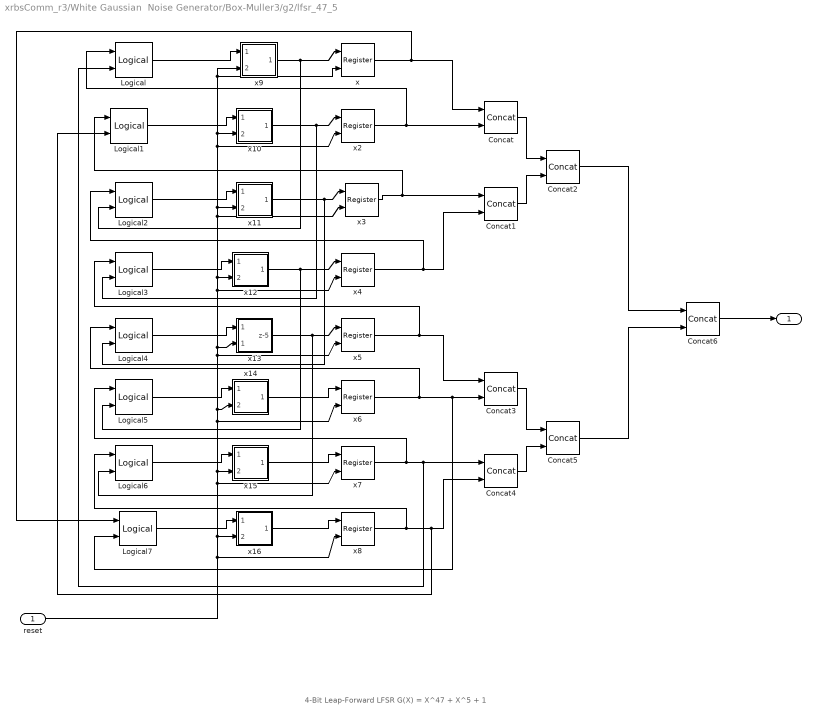
== system xrbsComm_r3/White Gaussian  Noise Generator/Box-Muller3/g2/lfsr_47_5 ==
  note: 4-Bit Leap-Forward LFSR G(X) = X^47 + X^5 + 1
  reset : Inport
  Concat{,1..6} (7 alike) : xbsIndex_r3/Concat  explicit_period=off  period=1  dbl_ovrd=off
  Logical{,1..7} (8 alike) : xbsIndex_r3/Logical  logical_function=XOR  inputs=2  precision=User Defined  arith_type=Unsigned  n_bits=1  bin_pt=0  align_bp=on  latency=0  explicit_period=on  period=-1  en=off  dbl_ovrd=off
      settings: xl_area=[0, 0, 0, 0, 0, 0, 0]
  x : xbsIndex_r3/Register  init=init(1)  reg_only_valid=off  explicit_period=off  period=1  rst=on  en=off  out_en=off  dbl_ovrd=off
      settings: xl_area=[0, 0, 0, 0, 0, 0, 0]
  x10 : Subsystem  mask{init=init(10:8:42)}
  x11 : Subsystem  mask{init=init(11:8:43)}
  x12 : Subsystem  mask{init=init(12:8:44)}
  x13 : Subsystem  mask{init=init(13:8:45)}
  x14 : Subsystem  mask{init=init(14:8:46)}
  x15 : Subsystem  mask{init=init(15:8:47)}
  x16 : Subsystem  mask{init=init(16:8:40)}
  x2 : xbsIndex_r3/Register  init=init(2)  reg_only_valid=off  explicit_period=off  period=1  rst=on  en=off  out_en=off  dbl_ovrd=off
      settings: xl_area=[0, 0, 0, 0, 0, 0, 0]
  x3 : xbsIndex_r3/Register  init=init(3)  reg_only_valid=off  explicit_period=off  period=1  rst=on  en=off  out_en=off  dbl_ovrd=off
      settings: xl_area=[0, 0, 0, 0, 0, 0, 0]
  x4 : xbsIndex_r3/Register  init=init(4)  reg_only_valid=off  explicit_period=off  period=1  rst=on  en=off  out_en=off  dbl_ovrd=off
      settings: xl_area=[0, 0, 0, 0, 0, 0, 0]
  x5 : xbsIndex_r3/Register  init=init(5)  reg_only_valid=off  explicit_period=off  period=1  rst=on  en=off  out_en=off  dbl_ovrd=off
      settings: xl_area=[0, 0, 0, 0, 0, 0, 0]
  x6 : xbsIndex_r3/Register  init=init(6)  reg_only_valid=off  explicit_period=off  period=1  rst=on  en=off  out_en=off  dbl_ovrd=off
      settings: xl_area=[0, 0, 0, 0, 0, 0, 0]
  x7 : xbsIndex_r3/Register  init=init(7)  reg_only_valid=off  explicit_period=off  period=1  rst=on  en=off  out_en=off  dbl_ovrd=off
      settings: xl_area=[0, 0, 0, 0, 0, 0, 0]
  x8 : xbsIndex_r3/Register  init=init(8)  reg_only_valid=off  explicit_period=off  period=1  rst=on  en=off  out_en=off  dbl_ovrd=off
      settings: xl_area=[0, 0, 0, 0, 0, 0, 0]
  x9 : Subsystem  mask{init=init(9:8:41)}
  " " : Outport
  wires:
  Logical/1 -> x9/1(" ")
  x9/1(z-5) -> x/1, Logical2/2
  x/1 -> Concat/1, Logical7/1
  x2/1 -> Concat/2, Logical/1
  Concat/1 -> Concat2/1
  x3/1 -> Concat1/1, Logical1/1
  x4/1 -> Concat1/2, Logical2/1
  Concat1/1 -> Concat2/2
  Logical1/1 -> x10/1("  ")
  x10/1(z-5) -> x2/1, Logical3/2
  Logical2/1 -> x11/1(" ")
  x11/1(z-5) -> x3/1, Logical4/2
  Logical3/1 -> x12/1(" ")
  x12/1(z-5) -> x4/1, Logical5/2
  Logical4/1 -> x13/1(" ")
  x13/1(z-5) -> x5/1, Logical6/2
  Logical5/1 -> x14/1(" ")
  x14/1(z-5) -> x6/1
  Logical6/1 -> x15/1(" ")
  x15/1(z-5) -> x7/1
  Logical7/1 -> x16/1(" ")
  x16/1(z-4) -> x8/1
  x6/1 -> Logical4/1, Concat3/2, Logical7/2
  Concat3/1 -> Concat5/1
  Concat4/1 -> Concat5/2
  x5/1 -> Concat3/1, Logical3/1
  x7/1 -> Concat4/1, Logical/2, Logical5/1
  x8/1 -> Concat4/2, Logical1/2, Logical6/1
  Concat2/1 -> Concat6/1
  Concat5/1 -> Concat6/2
  Concat6/1 -> " "/1
  reset/1 -> x9/2(reset), x/2, x10/2(reset), x2/2, x11/2(reset), x3/2, x12/2(reset), x4/2, x13/2(" 1"), x5/2, x14/2(reset), x6/2, x15/2(reset), x7/2, x16/2(reset), x8/2

== system xrbsComm_r3/White Gaussian  Noise Generator/Box-Muller4/fr1/iszero ==
  " " : Inport
  "const " : xbsIndex_r3/Constant  const=0  arith_type=Unsigned  n_bits=4  bin_pt=0  explicit_period=off  period=1  dbl_ovrd=off
  sel1 : xbsIndex_r3/Relational  mode=a=b  latency=1  explicit_period=off  period=1  en=off  dbl_ovrd=off
      settings: xl_area=[0, 0, 0, 0, 0, 0, 0]
  eq : Outport
  wires:
  "const "/1 -> sel1/2
  " "/1 -> sel1/1
  sel1/1 -> eq/1

== system xrbsComm_r3/White Gaussian  Noise Generator/Box-Muller4/fr1/iszero1 ==
  " " : Inport
  Constant1 : xbsIndex_r3/Constant  const=0  arith_type=Unsigned  n_bits=4  bin_pt=0  explicit_period=off  period=1  dbl_ovrd=off
  sel2 : xbsIndex_r3/Relational  mode=a=b  latency=1  explicit_period=off  period=1  en=off  dbl_ovrd=off
      settings: xl_area=[0, 0, 0, 0, 0, 0, 0]
  eq : Outport
  wires:
  Constant1/1 -> sel2/2
  " "/1 -> sel2/1
  sel2/1 -> eq/1

== system xrbsComm_r3/White Gaussian  Noise Generator/Box-Muller4/fr1/iszero2 ==
  " " : Inport
  Constant3 : xbsIndex_r3/Constant  const=0  arith_type=Unsigned  n_bits=4  bin_pt=0  explicit_period=off  period=1  dbl_ovrd=off
  sel3 : xbsIndex_r3/Relational  mode=a=b  latency=1  explicit_period=off  period=1  en=off  dbl_ovrd=off
      settings: xl_area=[0, 0, 0, 0, 0, 0, 0]
  eq : Outport
  wires:
  Constant3/1 -> sel3/2
  " "/1 -> sel3/1
  sel3/1 -> eq/1

== system xrbsComm_r3/White Gaussian  Noise Generator/Box-Muller4/fr1/iszero3 ==
  " " : Inport
  Constant : xbsIndex_r3/Constant  const=0  arith_type=Unsigned  n_bits=4  bin_pt=0  explicit_period=off  period=1  dbl_ovrd=off
  sel4 : xbsIndex_r3/Relational  mode=a=b  latency=1  explicit_period=off  period=1  en=off  dbl_ovrd=off
      settings: xl_area=[0, 0, 0, 0, 0, 0, 0]
  eq : Outport
  wires:
  Constant/1 -> sel4/2
  " "/1 -> sel4/1
  sel4/1 -> eq/1

== system xrbsComm_r3/White Gaussian  Noise Generator/Box-Muller4/fr1/lfsr_17_2 ==
  note: 4-Bit Leap-Forward LFSR G(X) = X^17 + X^3 + 1
  reset : Inport
  Concat : xbsIndex_r3/Concat  explicit_period=off  period=1  dbl_ovrd=off
  Concat1 : xbsIndex_r3/Concat  explicit_period=off  period=1  dbl_ovrd=off
  Concat2 : xbsIndex_r3/Concat  explicit_period=off  period=1  dbl_ovrd=off
  Logical{,1..3} (4 alike) : xbsIndex_r3/Logical  logical_function=XOR  inputs=2  precision=User Defined  arith_type=Unsigned  n_bits=1  bin_pt=0  align_bp=on  latency=0  explicit_period=on  period=-1  en=off  dbl_ovrd=off
      settings: xl_area=[0, 0, 0, 0, 0, 0, 0]
  x : xbsIndex_r3/Register  init=init(1)  reg_only_valid=off  explicit_period=off  period=1  rst=on  en=off  out_en=off  dbl_ovrd=off
      settings: xl_area=[0, 0, 0, 0, 0, 0, 0]
  x1 : Subsystem  mask{init=init(7:4:15)}
  x2 : xbsIndex_r3/Register  init=init(2)  reg_only_valid=off  explicit_period=off  period=1  rst=on  en=off  out_en=off  dbl_ovrd=off
      settings: xl_area=[0, 0, 0, 0, 0, 0, 0]
  x3 : xbsIndex_r3/Register  init=init(3)  reg_only_valid=off  explicit_period=off  period=1  rst=on  en=off  out_en=off  dbl_ovrd=off
      settings: xl_area=[0, 0, 0, 0, 0, 0, 0]
  x4 : xbsIndex_r3/Register  init=init(4)  reg_only_valid=off  explicit_period=off  period=1  rst=on  en=off  out_en=off  dbl_ovrd=off
      settings: xl_area=[0, 0, 0, 0, 0, 0, 0]
  x5 : Subsystem  mask{init=init(5:4:17)}
  x6 : Subsystem  mask{init=init(6:4:14)}
  x7 : Subsystem  mask{init=init(8:4:16)}
  " " : Outport
  wires:
  Logical/1 -> x5/1(" ")
  Logical1/1 -> x6/1(" ")
  Logical2/1 -> x1/1(" ")
  Logical3/1 -> x7/1(" ")
  x5/1(z-4) -> x/1, Logical2/2
  x6/1(z-3) -> x2/1, Logical3/2
  x1/1(z-3) -> x3/1, Logical/2
  x7/1(z-3) -> x4/1
  x/1 -> Logical1/1, Concat/1
  x2/1 -> Concat/2, Logical2/1
  Concat/1 -> Concat2/1
  x3/1 -> Concat1/1, Logical3/1
  x4/1 -> Concat1/2, Logical1/2, Logical/1
  Concat1/1 -> Concat2/2
  Concat2/1 -> " "/1
  reset/1 -> x5/2(reset), x6/2(" reset"), x1/2(" reset"), x7/2(reset), x/2, x2/2, x3/2, x4/2

== system xrbsComm_r3/White Gaussian  Noise Generator/Box-Muller4/fr1/lfsr_25_2 ==
  note: 4-Bit Leap-Forward LFSR G(X) = X^25 + X^3 + 1
  " reset" : Inport
  Concat : xbsIndex_r3/Concat  explicit_period=off  period=1  dbl_ovrd=off
  Concat1 : xbsIndex_r3/Concat  explicit_period=off  period=1  dbl_ovrd=off
  Concat2 : xbsIndex_r3/Concat  explicit_period=off  period=1  dbl_ovrd=off
  Logical{,1..3} (4 alike) : xbsIndex_r3/Logical  logical_function=XOR  inputs=2  precision=User Defined  arith_type=Unsigned  n_bits=1  bin_pt=0  align_bp=on  latency=0  explicit_period=on  period=-1  en=off  dbl_ovrd=off
      settings: xl_area=[0, 0, 0, 0, 0, 0, 0]
  x : xbsIndex_r3/Register  init=init(1)  reg_only_valid=off  explicit_period=off  period=1  rst=on  en=off  out_en=off  dbl_ovrd=off
      settings: xl_area=[0, 0, 0, 0, 0, 0, 0]
  x1 : Subsystem  mask{init=init(7:4:23)}
  x2 : xbsIndex_r3/Register  init=init(2)  reg_only_valid=off  explicit_period=off  period=1  rst=on  en=off  out_en=off  dbl_ovrd=off
      settings: xl_area=[0, 0, 0, 0, 0, 0, 0]
  x3 : xbsIndex_r3/Register  init=init(3)  reg_only_valid=off  explicit_period=off  period=1  rst=on  en=off  out_en=off  dbl_ovrd=off
      settings: xl_area=[0, 0, 0, 0, 0, 0, 0]
  x4 : xbsIndex_r3/Register  init=init(4)  reg_only_valid=off  explicit_period=off  period=1  rst=on  en=off  out_en=off  dbl_ovrd=off
      settings: xl_area=[0, 0, 0, 0, 0, 0, 0]
  x5 : Subsystem  mask{init=init(5:4:25)}
  x6 : Subsystem  mask{init=init(6:4:22)}
  x7 : Subsystem  mask{init=init(8:4:24)}
  " " : Outport
  wires:
  Concat2/1 -> " "/1
  Concat1/1 -> Concat2/2
  x4/1 -> Logical/1, Logical1/2, Concat1/2
  x3/1 -> Logical3/1, Concat1/1
  Concat/1 -> Concat2/1
  x2/1 -> Logical2/1, Concat/2
  x/1 -> Concat/1, Logical1/1
  x7/1(z-5) -> x4/1
  x1/1(z-5) -> Logical/2, x3/1
  x6/1(z-5) -> Logical3/2, x2/1
  x5/1(z-6) -> Logical2/2, x/1
  Logical3/1 -> x7/1(" ")
  Logical2/1 -> x1/1(" ")
  Logical1/1 -> x6/1(" ")
  Logical/1 -> x5/1(" ")
  " reset"/1 -> x7/2(reset), x1/2(reset), x6/2(reset), x5/2(reset), x/2, x2/2, x3/2, x4/2

== system xrbsComm_r3/White Gaussian  Noise Generator/Box-Muller4/fr1/lfsr_29_2 ==
  note: 4-Bit Leap-Forward LFSR G(X) = X^29 + X^2 + 1
  reset : Inport
  Concat : xbsIndex_r3/Concat  explicit_period=off  period=1  dbl_ovrd=off
  Concat1 : xbsIndex_r3/Concat  explicit_period=off  period=1  dbl_ovrd=off
  Concat2 : xbsIndex_r3/Concat  explicit_period=off  period=1  dbl_ovrd=off
  Logical{,1..3} (4 alike) : xbsIndex_r3/Logical  logical_function=XOR  inputs=2  precision=User Defined  arith_type=Unsigned  n_bits=1  bin_pt=0  align_bp=on  latency=0  explicit_period=on  period=-1  en=off  dbl_ovrd=off
      settings: xl_area=[0, 0, 0, 0, 0, 0, 0]
  x : xbsIndex_r3/Register  init=init(1)  reg_only_valid=off  explicit_period=off  period=1  rst=on  en=off  out_en=off  dbl_ovrd=off
      settings: xl_area=[0, 0, 0, 0, 0, 0, 0]
  x2 : xbsIndex_r3/Register  init=init(2)  reg_only_valid=off  explicit_period=off  period=1  rst=on  en=off  out_en=off  dbl_ovrd=off
      settings: xl_area=[0, 0, 0, 0, 0, 0, 0]
  x3 : xbsIndex_r3/Register  init=init(3)  reg_only_valid=off  explicit_period=off  period=1  rst=on  en=off  out_en=off  dbl_ovrd=off
      settings: xl_area=[0, 0, 0, 0, 0, 0, 0]
  x4 : xbsIndex_r3/Register  init=init(4)  reg_only_valid=off  explicit_period=off  period=1  rst=on  en=off  out_en=off  dbl_ovrd=off
      settings: xl_area=[0, 0, 0, 0, 0, 0, 0]
  x5 : Subsystem  mask{init=init(5:4:29)}
  x6 : Subsystem  mask{init=init(6:4:26)}
  x7 : Subsystem  mask{init=init(7:4:27)}
  x8 : Subsystem  mask{init=init(8:4:28)}
  " " : Outport
  wires:
  Logical/1 -> x5/1(" ")
  Logical1/1 -> x6/1(" ")
  Logical2/1 -> x7/1(" ")
  Logical3/1 -> x8/1(" ")
  x5/1(z-7) -> x/1, Logical3/2
  x6/1(z-6) -> x2/1, Logical/2
  x7/1(z-6) -> x3/1
  x8/1(z-6) -> x4/1
  x/1 -> Logical1/1, Concat/1
  x2/1 -> Concat/2, Logical2/1
  Concat/1 -> Concat2/1
  x3/1 -> Concat1/1, Logical1/2, Logical3/1
  x4/1 -> Concat1/2, Logical2/2, Logical/1
  Concat1/1 -> Concat2/2
  Concat2/1 -> " "/1
  reset/1 -> x8/2(reset), x7/2(reset), x6/2(reset), x5/2(reset), x/2, x2/2, x3/2, x4/2

== system xrbsComm_r3/White Gaussian  Noise Generator/Box-Muller4/fr1/lfsr_31_2 ==
  note: 4-Bit Leap-Forward LFSR G(X) = X^31 + X^3 + 1
  reset : Inport
  Concat : xbsIndex_r3/Concat  explicit_period=off  period=1  dbl_ovrd=off
  Concat1 : xbsIndex_r3/Concat  explicit_period=off  period=1  dbl_ovrd=off
  Concat2 : xbsIndex_r3/Concat  explicit_period=off  period=1  dbl_ovrd=off
  Logical{,1..3} (4 alike) : xbsIndex_r3/Logical  logical_function=XOR  inputs=2  precision=User Defined  arith_type=Unsigned  n_bits=1  bin_pt=0  align_bp=on  latency=0  explicit_period=on  period=-1  en=off  dbl_ovrd=off
      settings: xl_area=[0, 0, 0, 0, 0, 0, 0]
  x : xbsIndex_r3/Register  init=init(1)  reg_only_valid=off  explicit_period=off  period=1  rst=on  en=off  out_en=off  dbl_ovrd=off
      settings: xl_area=[0, 0, 0, 0, 0, 0, 0]
  x2 : xbsIndex_r3/Register  init=init(2)  reg_only_valid=off  explicit_period=off  period=1  rst=on  en=off  out_en=off  dbl_ovrd=off
      settings: xl_area=[0, 0, 0, 0, 0, 0, 0]
  x3 : xbsIndex_r3/Register  init=init(3)  reg_only_valid=off  explicit_period=off  period=1  rst=on  en=off  out_en=off  dbl_ovrd=off
      settings: xl_area=[0, 0, 0, 0, 0, 0, 0]
  x4 : xbsIndex_r3/Register  init=init(4)  reg_only_valid=off  explicit_period=off  period=1  rst=on  en=off  out_en=off  dbl_ovrd=off
      settings: xl_area=[0, 0, 0, 0, 0, 0, 0]
  x5 : Subsystem  mask{init=init(5:4:29)}
  x6 : Subsystem  mask{init=init(6:4:30)}
  x7 : Subsystem  mask{init=init(7:4:31)}
  x8 : Subsystem  mask{init=init(8:4:28)}
  " " : Outport
  wires:
  Logical/1 -> x5/1(" ")
  Logical1/1 -> x6/1(" ")
  Logical2/1 -> x7/1(" ")
  Logical3/1 -> x8/1(" ")
  x5/1(z-7) -> Logical/1, x/1
  x6/1(z-7) -> Logical1/1, x2/1
  x7/1(z-7) -> x3/1, Logical2/1
  x8/1(z-6) -> x4/1
  x/1 -> Concat/1, Logical3/1
  x2/1 -> Concat/2, Logical/2
  Concat/1 -> Concat2/1
  x3/1 -> Concat1/1, Logical1/2
  x4/1 -> Logical2/2, Concat1/2, Logical3/2
  Concat1/1 -> Concat2/2
  Concat2/1 -> " "/1
  reset/1 -> x5/2(reset), x6/2(reset), x7/2(reset), x8/2(reset), x/2, x2/2, x3/2, x4/2

== system xrbsComm_r3/White Gaussian  Noise Generator/Box-Muller4/fr1/lfsr_41_2 ==
  note: 4-Bit Leap-Forward LFSR G(X) = X^41 + X^3 + 1
  reset : Inport
  Concat : xbsIndex_r3/Concat  explicit_period=off  period=1  dbl_ovrd=off
  Concat1 : xbsIndex_r3/Concat  explicit_period=off  period=1  dbl_ovrd=off
  Concat2 : xbsIndex_r3/Concat  explicit_period=off  period=1  dbl_ovrd=off
  Logical{,1..3} (4 alike) : xbsIndex_r3/Logical  logical_function=XOR  inputs=2  precision=User Defined  arith_type=Unsigned  n_bits=1  bin_pt=0  align_bp=on  latency=0  explicit_period=on  period=-1  en=off  dbl_ovrd=off
      settings: xl_area=[0, 0, 0, 0, 0, 0, 0]
  x : xbsIndex_r3/Register  init=init(1)  reg_only_valid=off  explicit_period=off  period=1  rst=on  en=off  out_en=off  dbl_ovrd=off
      settings: xl_area=[0, 0, 0, 0, 0, 0, 0]
  x1 : Subsystem  mask{init=init(6:4:38)}
  x2 : xbsIndex_r3/Register  init=init(2)  reg_only_valid=off  explicit_period=off  period=1  rst=on  en=off  out_en=off  dbl_ovrd=off
      settings: xl_area=[0, 0, 0, 0, 0, 0, 0]
  x3 : xbsIndex_r3/Register  init=init(3)  reg_only_valid=off  explicit_period=off  period=1  rst=on  en=off  out_en=off  dbl_ovrd=off
      settings: xl_area=[0, 0, 0, 0, 0, 0, 0]
  x4 : xbsIndex_r3/Register  init=init(4)  reg_only_valid=off  explicit_period=off  period=1  rst=on  en=off  out_en=off  dbl_ovrd=off
      settings: xl_area=[0, 0, 0, 0, 0, 0, 0]
  x5 : Subsystem  mask{init=init(5:4:41)}
  x6 : Subsystem  mask{init=init(7:4:39)}
  x7 : Subsystem  mask{init=init(8:4:40)}
  " " : Outport
  wires:
  Logical/1 -> x5/1(" ")
  Logical1/1 -> x1/1(" ")
  Logical2/1 -> x6/1(" ")
  Logical3/1 -> x7/1(" ")
  x5/1(z-10) -> x/1, Logical2/2
  x1/1(z-9) -> x2/1, Logical3/2
  x6/1(z-9) -> x3/1, Logical/2
  x7/1(z-9) -> x4/1
  x/1 -> Logical1/1, Concat/1
  x2/1 -> Concat/2, Logical2/1
  Concat/1 -> Concat2/1
  x3/1 -> Concat1/1, Logical3/1
  x4/1 -> Concat1/2, Logical1/2, Logical/1
  Concat1/1 -> Concat2/2
  Concat2/1 -> " "/1
  reset/1 -> x5/2(reset), x1/2(reset), x6/2(reset), x7/2(reset), x/2, x2/2, x3/2, x4/2
